simulink model "HW02_Q2_Bishop"  (R2022a)
settings: Solver=VariableStepAuto  StartTime=0.0  StopTime=10.0  RelTol=1e-3
libraries: dspsrcs4 x1
settings Model: Creator=ebishop  LastModifiedBy=ebishop

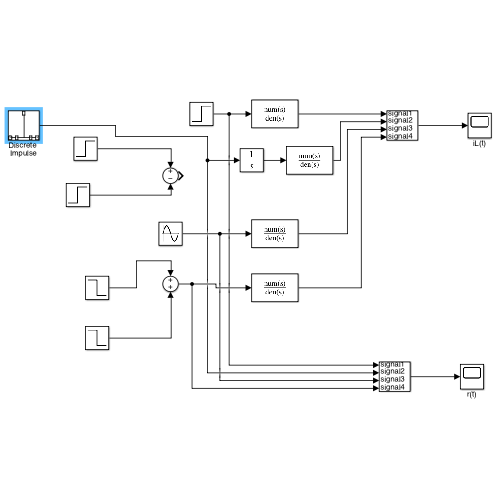
[thumbnail: Simulink's stored preview of the top-level diagram]
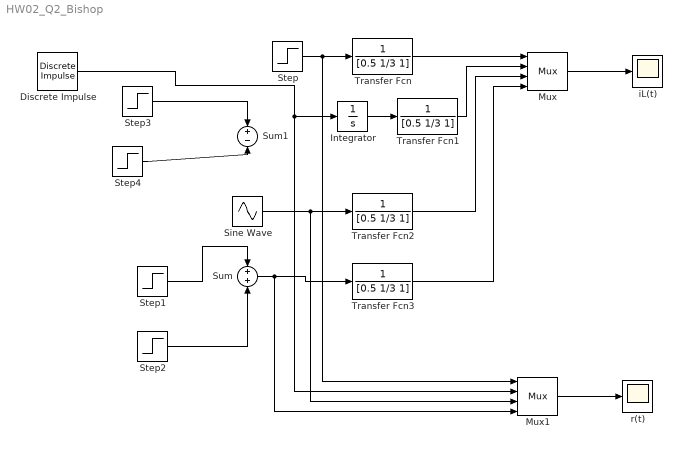
== system HW02_Q2_Bishop ==
  Discrete Impulse : dspsrcs4/Discrete  Impulse  Delay=0  SampleTime=1  FrameSample=1  OutputFrames=off  dataType=double  isSigned=on  wordLen=16  udDataType=sfix(16)  fracBitsMode=Best precision  numFracBits=15  OutDataTypeStr=double  LastOutDataTypeStr=double
  Integrator : Integrator
  Mux : Mux
      settings: DisplayOption=signals
  Mux1 : Mux
      settings: DisplayOption=signals
  Sine Wave : Sin  SampleTime=0
  Step : Step  Time=0  SampleTime=0
  Step1 : Step  Time=0  Before=1  After=0  SampleTime=0
  Step2 : Step  Time=2  Before=1  After=0  SampleTime=0
  Step3 : Step  Time=0.025  SampleTime=0
  Step4 : Step  Time=0.05  SampleTime=0
  Sum : Sum
  Sum1 : Sum  Inputs=+-
  Transfer Fcn{,1..3} (4 alike) : TransferFcn  Denominator=[0.5 1/3 1]
  iL(t) : Scope
  r(t) : Scope
  wires:
  Mux/1 -> iL(t)/1
  Step/1 -> Mux1/1, Transfer Fcn/1
  Sine Wave/1 -> Mux1/3, Transfer Fcn2/1
  Transfer Fcn/1 -> Mux/1
  Transfer Fcn2/1 -> Mux/3
  Transfer Fcn3/1 -> Mux/4
  Step1/1 -> Sum/1
  Sum/1 -> Mux1/4, Transfer Fcn3/1
  Step2/1 -> Sum/2
  Mux1/1 -> r(t)/1
  Step4/1 -> Sum1/2
  Step3/1 -> Sum1/1
  Discrete Impulse/1 -> Integrator/1, Mux1/2
  Integrator/1 -> Transfer Fcn1/1
  Transfer Fcn1/1 -> Mux/2
